simulink model "sawtooth_triangular"  (R2024b)
settings: Solver=VariableStepAuto  StartTime=0.0  StopTime=10.0  RelTol=1e-3
libraries: simulink x3
settings Model: Creator=sanja  LastModifiedBy=sanja

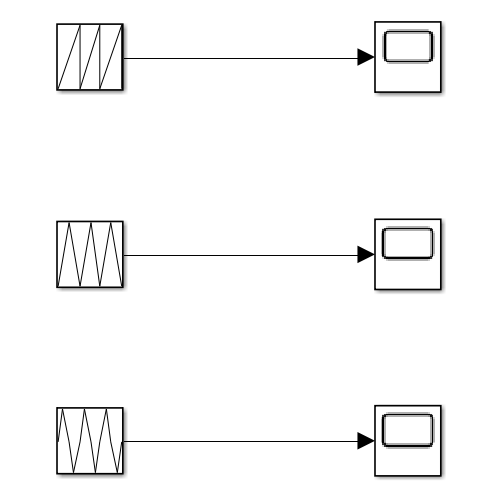
[thumbnail: Simulink's stored preview of the top-level diagram]
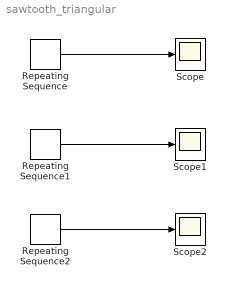
== system sawtooth_triangular ==
  Repeating Sequence : simulink/Sources/Repeating Sequence  rep_seq_t=[0 2]  rep_seq_y=[0 5]
  Repeating Sequence1 : simulink/Sources/Repeating Sequence  rep_seq_t=[0 1 2]  rep_seq_y=[0 5 0]
  Repeating Sequence2 : simulink/Sources/Repeating Sequence  rep_seq_t=[0 0.02/4 0.02/2 0.02*3/4 0.02]  rep_seq_y=[0 1 0 -1 0]
  Scope : Scope
  Scope1 : Scope
  Scope2 : Scope
  wires:
  Repeating Sequence/1 -> Scope/1
  Repeating Sequence1/1 -> Scope1/1
  Repeating Sequence2/1 -> Scope2/1
